simulink model "seguimiento_de_trayectoria"  (R2020b)
settings: Solver=ode5  StartTime=0.0  StopTime=inf  RelTol=1e-3
undefined symbols (not defined in the file): National_Instruments, PCI
libraries: sldrtlib x2, simulink x1
settings Model: SimulationMode=external  Creator=Usuario_UMA  LastModifiedBy=alumnoic06
settings RTWCC: Description=Simulink Desktop Real-Time  SystemTargetFile=sldrt.tlc  TemplateMakefile=sldrt.tmf  RTWCompilerOptimization=on
settings CodeAppCC: MaxIdLength=95
settings SimulinkDesktopRealTimeCC: TargetPreCompLibLocation=C:\Program Files\MATLAB\R2020\toolbox\sldrt\lib\win64

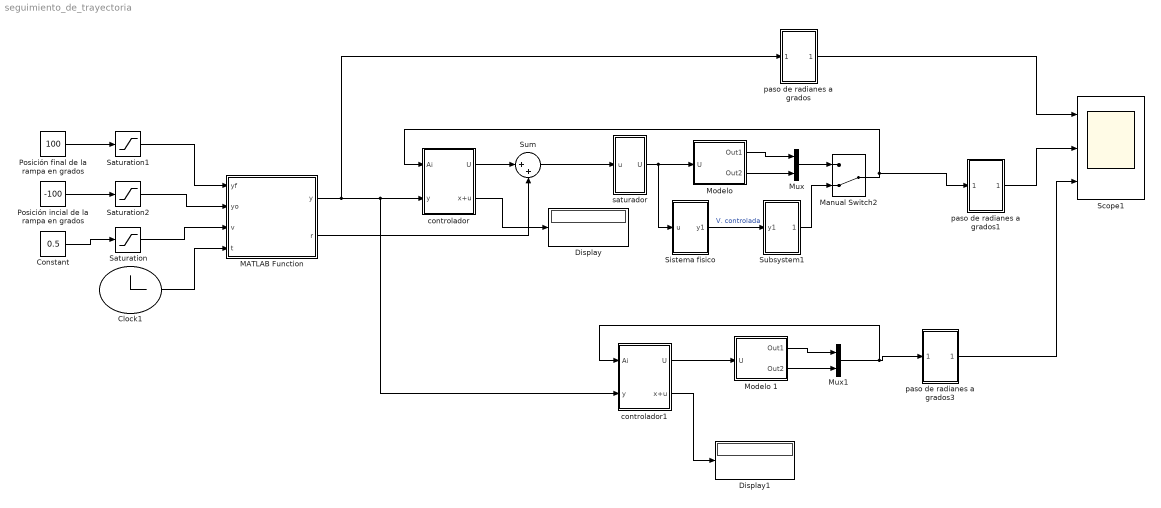
== system seguimiento_de_trayectoria ==
  Clock1 : Clock
      settings: Decimation=4
  Constant : Constant  Value=0.5
  Display : Display
  Display1 : Display
  MATLAB Function : MATLAB Function  TreatAsAtomicUnit=on
  Manual Switch2 : ManualSwitch  CurrentSetting=0
  "Modelo " : Subsystem
  Modelo 1 : Subsystem
  Mux : Mux  Inputs=2
  Mux1 : Mux  Inputs=2
  Posición final de la rampa en grados : Constant  Value=100
  Posición incial de la rampa en grados : Constant  Value=-100
  Saturation : Saturate  UpperLimit=4.7  LowerLimit=-4.7
  Saturation1 : Saturate  UpperLimit=100  LowerLimit=-100
  Saturation2 : Saturate  UpperLimit=100  LowerLimit=-100
  Scope1 : Scope  NumInputPorts=3
  Sistema fisico : Subsystem
  Subsystem1 : Subsystem
  Sum : Sum  Inputs=|++
  controlador : Subsystem
  controlador1 : Subsystem
  paso de radianes a grados : Subsystem
  paso de radianes a grados1 : Subsystem
  paso de radianes a grados3 : Subsystem
  saturador : Subsystem
  wires:
  paso de radianes a grados/1(Out1) -> Scope1/1
  Sistema fisico/1(y1) -> Subsystem1/1(y1)  "V. controlada"
  MATLAB Function/1(y) -> paso de radianes a grados/1(In1), controlador1/2(y), controlador/2(y)
  Posición final de la rampa en grados/1 -> Saturation1/1
  MATLAB Function/2(r) -> Sum/2
  paso de radianes a grados1/1(Out1) -> Scope1/2
  Constant/1 -> Saturation/1
  Sum/1 -> saturador/1(u)
  Saturation1/1 -> MATLAB Function/1(yf)
  Saturation2/1 -> MATLAB Function/2(yo)
  Posición incial de la rampa en grados/1 -> Saturation2/1
  Saturation/1 -> MATLAB Function/3(v)
  controlador/2(x+u) -> Display/1
  "Modelo "/1(Out1) -> Mux/1
  "Modelo "/2(Out2) -> Mux/2
  Clock1/1 -> MATLAB Function/4(t)
  saturador/1(U) -> "Modelo "/1(U), Sistema fisico/1(u)
  controlador/1(U) -> Sum/1
  Mux/1 -> Manual Switch2/1
  Manual Switch2/1 -> controlador/1(Ai), paso de radianes a grados1/1(In1)
  Subsystem1/1(Out1) -> Manual Switch2/2
  Modelo 1/2(Out2) -> Mux1/2
  Mux1/1 -> controlador1/1(Ai), paso de radianes a grados3/1(In1)
  Modelo 1/1(Out1) -> Mux1/1
  controlador1/1(U) -> Modelo 1/1(U)
  paso de radianes a grados3/1(Out1) -> Scope1/3
  controlador1/2(x+u) -> Display1/1

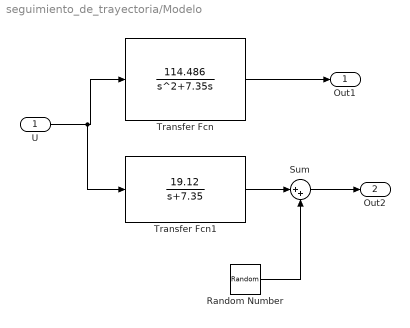
== system seguimiento_de_trayectoria/Modelo  ==
  U : Inport
  Random Number : RandomNumber  Variance=0  SampleTime=0
  Sum : Sum  Inputs=|++
  Transfer Fcn : TransferFcn  Numerator=[114.486]  Denominator=[1 7.35 0]
  Transfer Fcn1 : TransferFcn  Numerator=[19.12]  Denominator=[1 7.35]
  Out1 : Outport
  Out2 : Outport  Port=2
  wires:
  U/1 -> Transfer Fcn1/1, Transfer Fcn/1
  Transfer Fcn/1 -> Out1/1
  Transfer Fcn1/1 -> Sum/1
  Random Number/1 -> Sum/2
  Sum/1 -> Out2/1

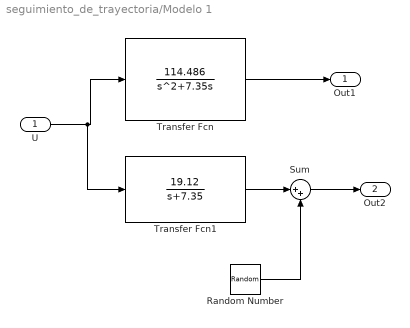
== system seguimiento_de_trayectoria/Modelo 1 ==
  U : Inport
  Random Number : RandomNumber  Variance=0  SampleTime=0
  Sum : Sum  Inputs=|++
  Transfer Fcn : TransferFcn  Numerator=[114.486]  Denominator=[1 7.35 0]
  Transfer Fcn1 : TransferFcn  Numerator=[19.12]  Denominator=[1 7.35]
  Out1 : Outport
  Out2 : Outport  Port=2
  wires:
  U/1 -> Transfer Fcn1/1, Transfer Fcn/1
  Transfer Fcn/1 -> Out1/1
  Transfer Fcn1/1 -> Sum/1
  Random Number/1 -> Sum/2
  Sum/1 -> Out2/1

== system seguimiento_de_trayectoria/Sistema fisico ==
  u : Inport
  Analog Input2 : sldrtlib/Analog Input  SampleTime=0.001  MaxMissedTicks=10  ShowMissedTicks=off  YieldWhenWaiting=off  DrvName=National_Instruments/PCI-6014  DrvAddress=4294967295  DrvOptions=[2 0 0 0 0 0]  Channels=[1,2]  RangeMode=1  VoltRange=1  DataType=1
      settings: AttributesFormatString=National Instruments\nPCI-6014 [auto]
  Analog Output : sldrtlib/Analog Output  SampleTime=0.001  MaxMissedTicks=10  ShowMissedTicks=off  YieldWhenWaiting=off  DrvName=National_Instruments/PCI-6014  DrvAddress=4294967295  DrvOptions=[2 0 0 0 0 0]  Channels=1  RangeMode=1  VoltRange=1  InitialValue=[]  FinalValue=[]
      settings: AttributesFormatString=National Instruments\nPCI-6014 [auto]
  y1 : Outport
  wires:
  u/1 -> Analog Output/1
  Analog Input2/1 -> y1/1  "Original signal"

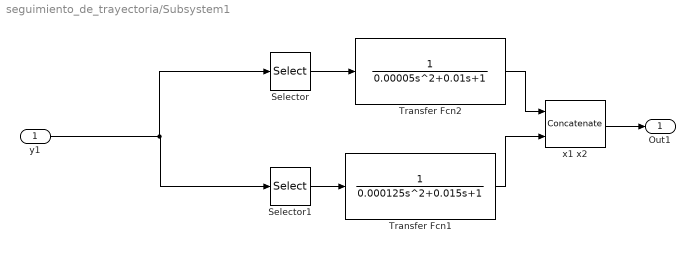
== system seguimiento_de_trayectoria/Subsystem1 ==
  y1 : Inport
  Selector : Selector  InputPortWidth=2  IndexOptions=Index vector (dialog)  Indices=[1]  OutputSizes=1
  Selector1 : Selector  InputPortWidth=2  IndexOptions=Index vector (dialog)  Indices=[2]  OutputSizes=1
  Transfer Fcn1 : TransferFcn  Denominator=[0.000125 0.015 1]
  Transfer Fcn2 : TransferFcn  Denominator=[0.00005 0.01 1]
  "x1 x2 " : Concatenate  ConcatenateDimension=2
  Out1 : Outport
  wires:
  Selector1/1 -> Transfer Fcn1/1
  "x1 x2 "/1 -> Out1/1
  y1/1 -> Selector/1, Selector1/1
  Transfer Fcn1/1 -> "x1 x2 "/2
  Selector/1 -> Transfer Fcn2/1
  Transfer Fcn2/1 -> "x1 x2 "/1

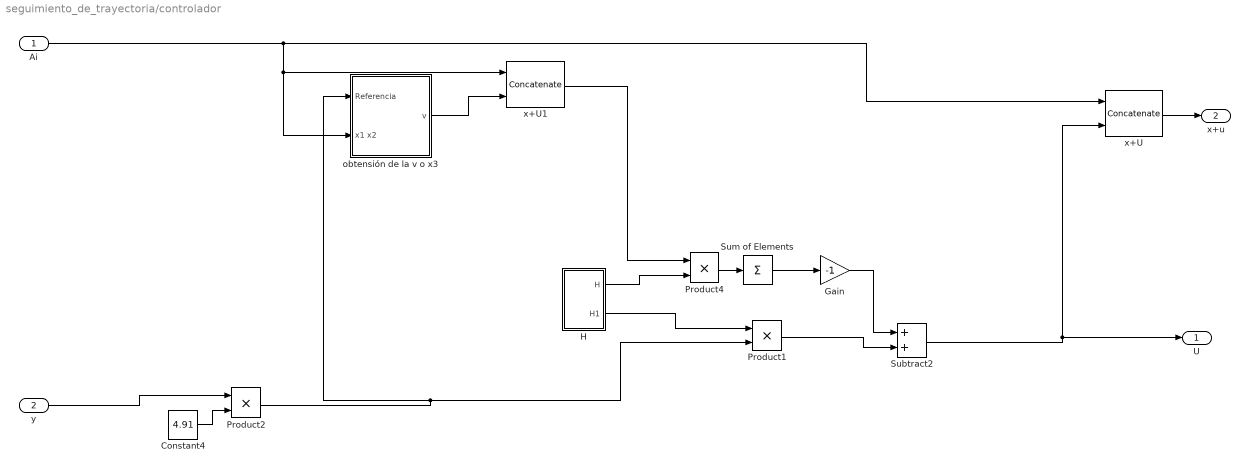
== system seguimiento_de_trayectoria/controlador ==
  Ai : Inport  OutDataTypeStr=double
  y : Inport  Port=2
  Constant4 : Constant  Value=4.91
  Gain : Gain  Gain=-1
  H : Subsystem  mask{h1=15.349, h2=0.75, h3=-0.019}
  Product1 : Product
  Product2 : Product
  Product4 : Product
  Subtract2 : Sum  OutDataTypeStr=double
  Sum of Elements : Sum  Inputs=+
  obtensión de la v o x3 : Subsystem
  x+U : Concatenate  ConcatenateDimension=2
  x+U1 : Concatenate  ConcatenateDimension=2
  U : Outport  OutDataTypeStr=double
  x+u : Outport  Port=2
  wires:
  Product4/1 -> Sum of Elements/1
  Gain/1 -> Subtract2/1
  Product2/1 -> obtensión de la v o x3/1(Referencia), Product1/2
  H/1(H) -> Product4/2
  H/2(H1) -> Product1/1
  Sum of Elements/1 -> Gain/1
  Product1/1 -> Subtract2/2
  x+U/1 -> x+u/1
  obtensión de la v o x3/1(v) -> x+U1/2
  x+U1/1 -> Product4/1
  Ai/1 -> x+U/1, obtensión de la v o x3/2(x1 x2), x+U1/1
  Constant4/1 -> Product2/2
  y/1 -> Product2/1
  Subtract2/1 -> x+U/2, U/1

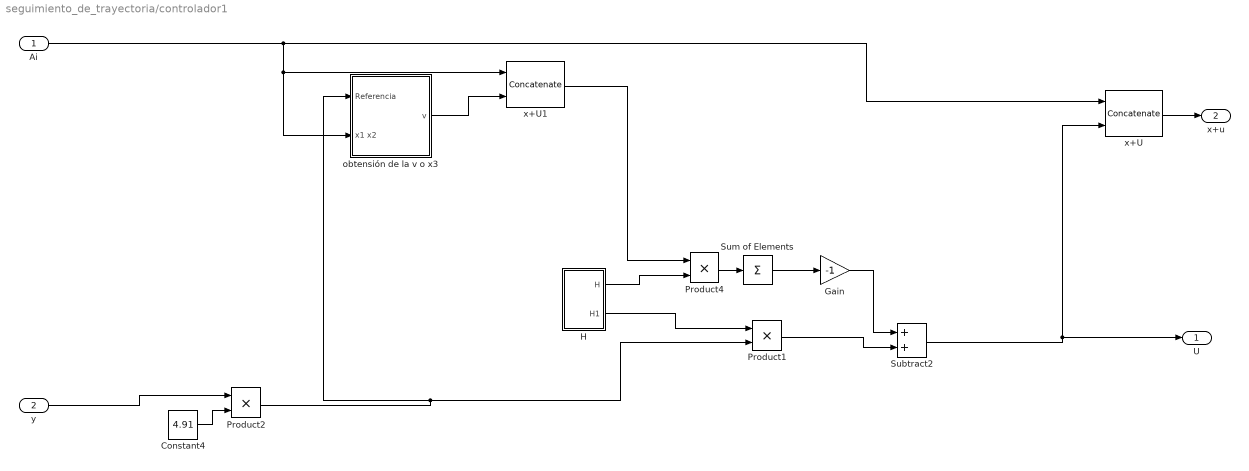
== system seguimiento_de_trayectoria/controlador1 ==
  Ai : Inport  OutDataTypeStr=double
  y : Inport  Port=2
  Constant4 : Constant  Value=4.91
  Gain : Gain  Gain=-1
  H : Subsystem  mask{h1=15.349, h2=0.75, h3=-0.019}
  Product1 : Product
  Product2 : Product
  Product4 : Product
  Subtract2 : Sum  OutDataTypeStr=double
  Sum of Elements : Sum  Inputs=+
  obtensión de la v o x3 : Subsystem
  x+U : Concatenate  ConcatenateDimension=2
  x+U1 : Concatenate  ConcatenateDimension=2
  U : Outport  OutDataTypeStr=double
  x+u : Outport  Port=2
  wires:
  Product4/1 -> Sum of Elements/1
  Gain/1 -> Subtract2/1
  Product2/1 -> obtensión de la v o x3/1(Referencia), Product1/2
  H/1(H) -> Product4/2
  H/2(H1) -> Product1/1
  Sum of Elements/1 -> Gain/1
  Product1/1 -> Subtract2/2
  x+U/1 -> x+u/1
  obtensión de la v o x3/1(v) -> x+U1/2
  x+U1/1 -> Product4/1
  Ai/1 -> x+U/1, obtensión de la v o x3/2(x1 x2), x+U1/1
  Constant4/1 -> Product2/2
  y/1 -> Product2/1
  Subtract2/1 -> x+U/2, U/1

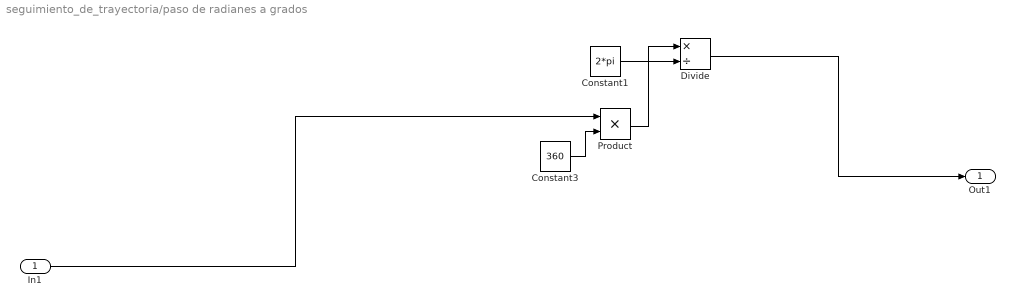
== system seguimiento_de_trayectoria/paso de radianes a grados ==
  In1 : Inport
  Constant1 : Constant  Value=2*pi
  Constant3 : Constant  Value=360
  Divide : Product  Inputs=*/
  Product : Product
  Out1 : Outport
  wires:
  Product/1 -> Divide/1
  Constant1/1 -> Divide/2
  Constant3/1 -> Product/2
  Divide/1 -> Out1/1
  In1/1 -> Product/1

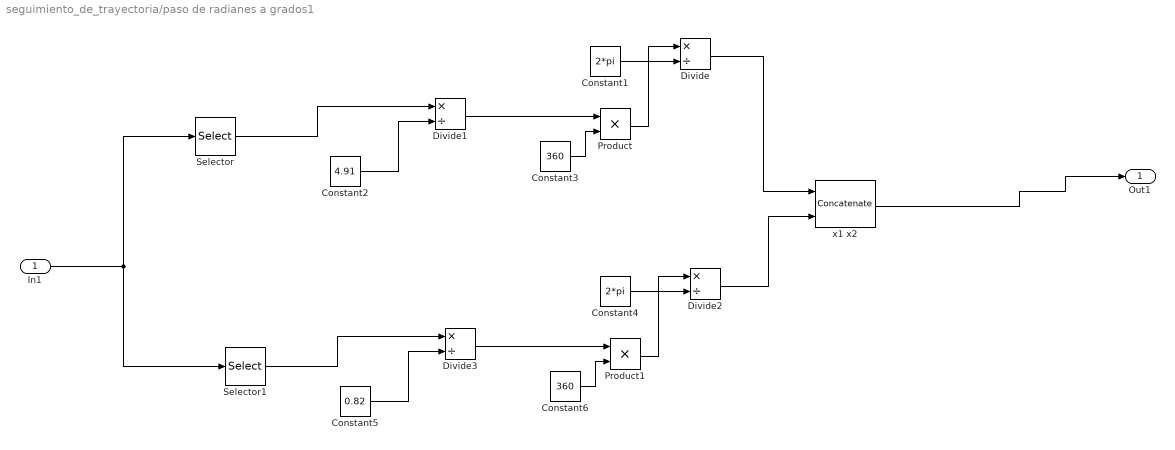
== system seguimiento_de_trayectoria/paso de radianes a grados1 ==
  In1 : Inport
  Constant1 : Constant  Value=2*pi
  Constant2 : Constant  Value=4.91
  Constant3 : Constant  Value=360
  Constant4 : Constant  Value=2*pi
  Constant5 : Constant  Value=0.82
  Constant6 : Constant  Value=360
  Divide{,1..3} (4 alike) : Product  Inputs=*/
  Product : Product
  Product1 : Product
  Selector : Selector  InputPortWidth=2  IndexOptions=Index vector (dialog)  Indices=[1]  OutputSizes=1
  Selector1 : Selector  InputPortWidth=2  IndexOptions=Index vector (dialog)  Indices=[2]  OutputSizes=1
  x1 x2 : Concatenate  ConcatenateDimension=2
  Out1 : Outport
  wires:
  Product/1 -> Divide/1
  Constant1/1 -> Divide/2
  Constant3/1 -> Product/2
  Divide1/1 -> Product/1
  Constant2/1 -> Divide1/2
  Selector/1 -> Divide1/1
  In1/1 -> Selector1/1, Selector/1
  Constant6/1 -> Product1/2
  Constant5/1 -> Divide3/2
  Constant4/1 -> Divide2/2
  Product1/1 -> Divide2/1
  Divide3/1 -> Product1/1
  Selector1/1 -> Divide3/1
  Divide2/1 -> x1 x2/2
  Divide/1 -> x1 x2/1
  x1 x2/1 -> Out1/1

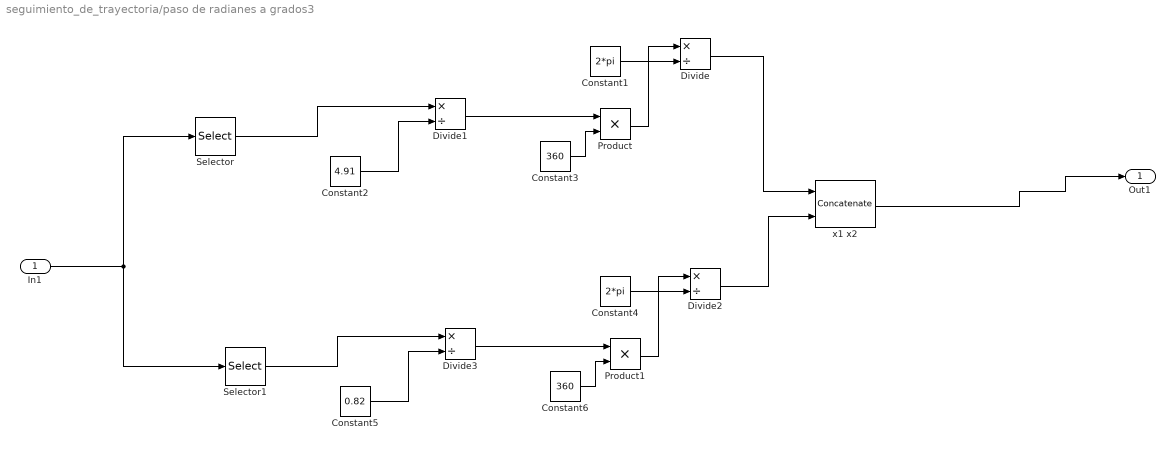
== system seguimiento_de_trayectoria/paso de radianes a grados3 ==
  In1 : Inport
  Constant1 : Constant  Value=2*pi
  Constant2 : Constant  Value=4.91
  Constant3 : Constant  Value=360
  Constant4 : Constant  Value=2*pi
  Constant5 : Constant  Value=0.82
  Constant6 : Constant  Value=360
  Divide{,1..3} (4 alike) : Product  Inputs=*/
  Product : Product
  Product1 : Product
  Selector : Selector  InputPortWidth=2  IndexOptions=Index vector (dialog)  Indices=[1]  OutputSizes=1
  Selector1 : Selector  InputPortWidth=2  IndexOptions=Index vector (dialog)  Indices=[2]  OutputSizes=1
  x1 x2 : Concatenate  ConcatenateDimension=2
  Out1 : Outport
  wires:
  Product/1 -> Divide/1
  Constant1/1 -> Divide/2
  Constant3/1 -> Product/2
  Divide1/1 -> Product/1
  Constant2/1 -> Divide1/2
  Selector/1 -> Divide1/1
  In1/1 -> Selector1/1, Selector/1
  Constant6/1 -> Product1/2
  Constant5/1 -> Divide3/2
  Constant4/1 -> Divide2/2
  Product1/1 -> Divide2/1
  Divide3/1 -> Product1/1
  Selector1/1 -> Divide3/1
  Divide2/1 -> x1 x2/2
  Divide/1 -> x1 x2/1
  x1 x2/1 -> Out1/1

== system seguimiento_de_trayectoria/saturador ==
  u : Inport  OutDataTypeStr=double
  Constant1 : Constant  Value=-5
  Constant2 : Constant  Value=5
  Saturation Dynamic : simulink/Discontinuities/Saturation Dynamic  OutMin=-5  OutMax=5  OutDataTypeStr=Inherit: Same as second input  OutDataType=fixdt(1, 16)  OutScaling=2^-10  DoSatur=off
  U : Outport  OutDataTypeStr=double
  wires:
  u/1 -> Saturation Dynamic/2
  Constant2/1 -> Saturation Dynamic/1
  Saturation Dynamic/1 -> U/1
  Constant1/1 -> Saturation Dynamic/3

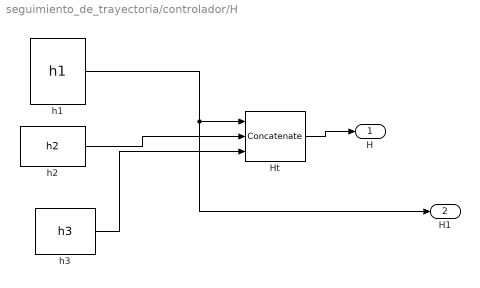
== system seguimiento_de_trayectoria/controlador/H ==
  Ht : Concatenate  NumInputs=3  ConcatenateDimension=2
  h1 : Constant  Value=h1
  h2 : Constant  Value=h2
  h3 : Constant  Value=h3
  H : Outport
  H1 : Outport  Port=2
  wires:
  h1/1 -> H1/1, Ht/1
  h2/1 -> Ht/2
  Ht/1 -> H/1
  h3/1 -> Ht/3

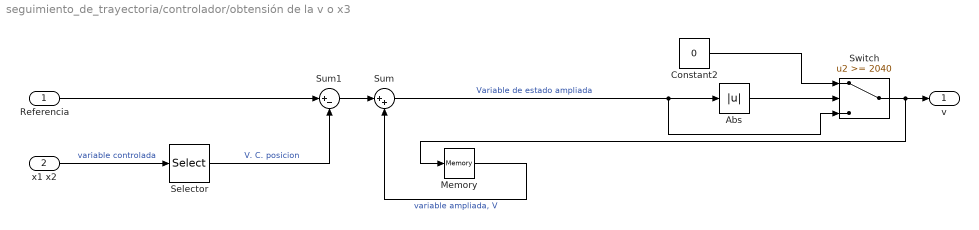
== system seguimiento_de_trayectoria/controlador/obtensión de la v o x3 ==
  Referencia : Inport
  x1 x2 : Inport  Port=2  PortDimensions=2
  Abs : Abs
  Constant2 : Constant  Value=0
  Memory : Memory  InheritSampleTime=on  LinearizeAsDelay=on
  Selector : Selector  InputPortWidth=2  IndexOptions=Index vector (dialog)  Indices=[1]  OutputSizes=1
  Sum : Sum  Inputs=|++
  Sum1 : Sum  Inputs=|+-
  Switch : Switch  Threshold=2040
  v : Outport
  wires:
  Referencia/1 -> Sum1/1
  Sum/1 -> Switch/3, Abs/1  "Variable de estado ampliada"
  Sum1/1 -> Sum/1
  Memory/1 -> Sum/2  "variable ampliada, V"
  x1 x2/1 -> Selector/1  "variable controlada"
  Selector/1 -> Sum1/2  "V. C. posicion"
  Constant2/1 -> Switch/1
  Abs/1 -> Switch/2
  Switch/1 -> Memory/1, v/1

== system seguimiento_de_trayectoria/controlador1/H ==
  Ht : Concatenate  NumInputs=3  ConcatenateDimension=2
  h1 : Constant  Value=h1
  h2 : Constant  Value=h2
  h3 : Constant  Value=h3
  H : Outport
  H1 : Outport  Port=2
  wires:
  h1/1 -> H1/1, Ht/1
  h2/1 -> Ht/2
  Ht/1 -> H/1
  h3/1 -> Ht/3

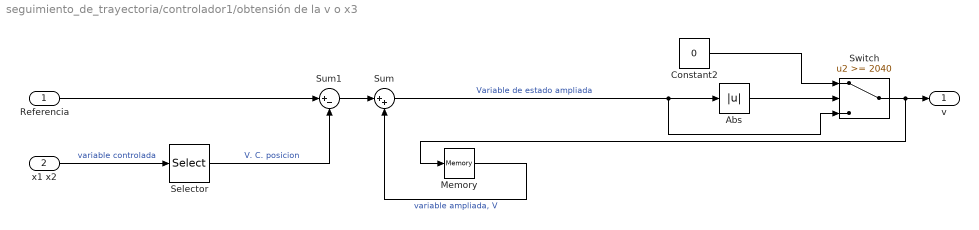
== system seguimiento_de_trayectoria/controlador1/obtensión de la v o x3 ==
  Referencia : Inport
  x1 x2 : Inport  Port=2  PortDimensions=2
  Abs : Abs
  Constant2 : Constant  Value=0
  Memory : Memory  InheritSampleTime=on  LinearizeAsDelay=on
  Selector : Selector  InputPortWidth=2  IndexOptions=Index vector (dialog)  Indices=[1]  OutputSizes=1
  Sum : Sum  Inputs=|++
  Sum1 : Sum  Inputs=|+-
  Switch : Switch  Threshold=2040
  v : Outport
  wires:
  Referencia/1 -> Sum1/1
  Sum/1 -> Switch/3, Abs/1  "Variable de estado ampliada"
  Sum1/1 -> Sum/1
  Memory/1 -> Sum/2  "variable ampliada, V"
  x1 x2/1 -> Selector/1  "variable controlada"
  Selector/1 -> Sum1/2  "V. C. posicion"
  Constant2/1 -> Switch/1
  Abs/1 -> Switch/2
  Switch/1 -> Memory/1, v/1

== matlab function seguimiento_de_trayectoria/MATLAB Function ==
  data: yf input; y output; yo input; v input; r output; t input
function[y,r]= fcn(yf,yo,v,t)
 yfr=(yf*2*pi/360);
 yor=(yo*2*pi/360);
tf=(yfr-yor)/v;

y=yor+v*t;
r=(7.35/114.486)*v;
if t>tf
   y=yfr
   
end

end
